simulink model "fuzzy_simulink_rise"  (R2015b)
settings: Solver=VariableStepAuto  StartTime=0.0  StopTime=200  RelTol=1e-3
libraries: fuzblock x1
settings Model: Creator=giorgos  LastModifiedBy=giorgos

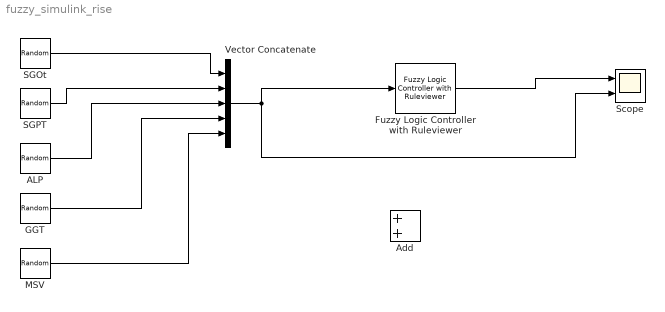
== system fuzzy_simulink_rise ==
  ALP : RandomNumber  Mean=60  Variance=0  SampleTime=5
  Add : Sum
  Fuzzy Logic Controller with Ruleviewer : fuzblock/Fuzzy Logic  Controller  with Ruleviewer  fismatrix=a  Ts=5
  GGT : RandomNumber  Mean=25  Variance=0  SampleTime=5
  MSV : RandomNumber  Mean=88  Variance=0  SampleTime=5
  "SGOt " : RandomNumber  Mean=15  Variance=0  SampleTime=5
  SGPT : RandomNumber  Mean=14  Variance=0  SampleTime=5
  Scope : Scope  NumInputPorts=2
  Vector Concatenate : Concatenate  NumInputs=5
  wires:
  MSV/1 -> Vector Concatenate/5
  GGT/1 -> Vector Concatenate/4
  "SGOt "/1 -> Vector Concatenate/1
  ALP/1 -> Vector Concatenate/3
  Vector Concatenate/1 -> Scope/2, Fuzzy Logic Controller with Ruleviewer/1
  SGPT/1 -> Vector Concatenate/2
  Fuzzy Logic Controller with Ruleviewer/1 -> Scope/1
